simulink model "model"  (R2024a)
settings: Solver=VariableStepAuto  StartTime=0.0  StopTime=80  RelTol=1e-3
values from neighbouring files (symbols this model uses):
  b = 0.5*CdA*rho    (= 0.3316545)    [init.m]    (also in stateFcnTaycan.m)
  F_max = [22000 1710]    [init.m]    (also in stateFcnTaycan.m = interp1(v_to_F_max_lu, F_max_lu, v, 'linear'))
  F_min = -20000    [init.m]    (also in stateFcnTaycan.m)
  g = 9.81    [init.m]
  m = 2140    [init.m]    (also in stateFcnTaycan.m)
  Ts = 1    [init.m]
  v_to_F_max = [0 72]    [init.m]
libraries: simulink x3, mpclib x1
settings Model: Creator=berto  LastModifiedBy=berto

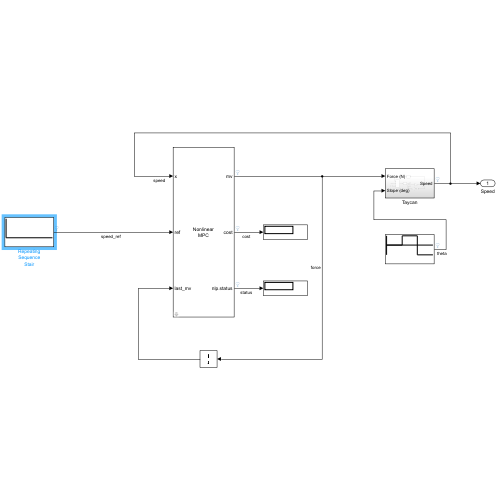
[thumbnail: Simulink's stored preview of the top-level diagram]
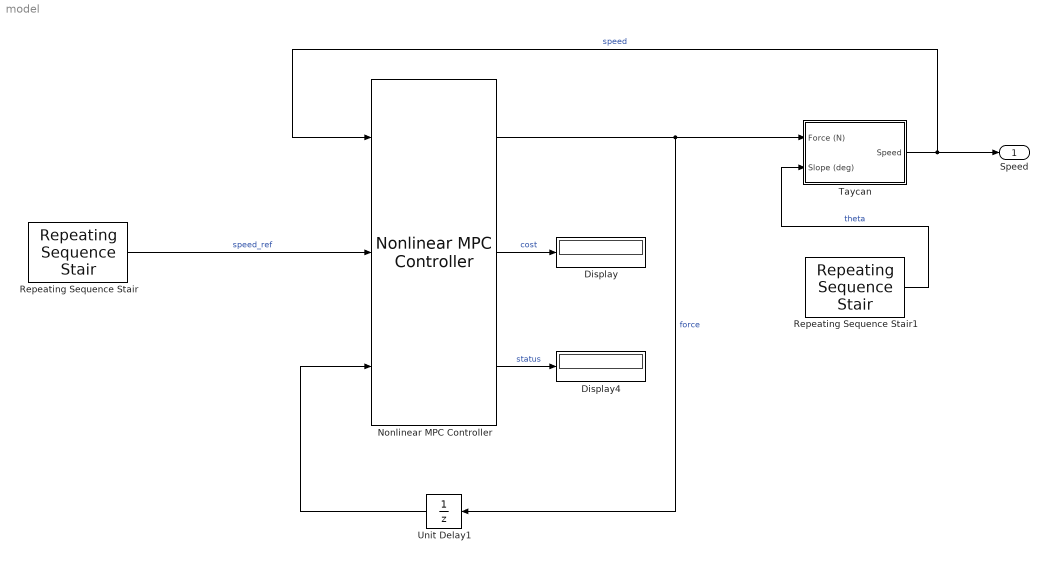
== system model ==
  Display : Display
  Display4 : Display
  Nonlinear MPC Controller : mpclib/Nonlinear MPC Controller  nlmpcobj=nlobj  UseObjectTs=on  UseMEX=off  md_enabled=off  mvtarget_enabled=off  param_enabled=off  cost_enabled=on  mvseq_enabled=off  stateseq_enabled=off  ovseq_enabled=off  slack_enabled=off  status_enabled=on  ov_min=off  ov_max=off  mv_min=off  mv_max=off  mvrate_min=off  mvrate_max=off  state_min=off  state_max=off  ov_weight=off  mv_weight=off  mvrate_weight=off  ecr_weight=off  nlp_initialize=off
  Repeating Sequence Stair : simulink/Sources/Repeating Sequence Stair  OutValues=40  tsamp=20  OutMin=[]  OutMax=[]  OutDataTypeStr=double  OutputDataTypeScalingMode=double  OutDataType=fixdt(0,8)  ConRadixGroup=Best Precision: Vector-wise  OutScaling=2^-12
  Repeating Sequence Stair1 : simulink/Sources/Repeating Sequence Stair  OutValues=[0 10 -10].'  tsamp=20  OutMin=[]  OutMax=[]  OutDataTypeStr=double  OutputDataTypeScalingMode=double  OutDataType=fixdt(0,8)  ConRadixGroup=Best Precision: Vector-wise  OutScaling=2^-12
  Taycan : Subsystem
  Unit Delay1 : UnitDelay  SampleTime=Ts  HasFrameUpgradeWarning=on
  Speed : Outport
  wires:
  Taycan/1(Speed) -> Nonlinear MPC Controller/1, Speed/1  "speed"
  Nonlinear MPC Controller/1 -> Taycan/1(Force (N)), Unit Delay1/1  "force"
  Repeating Sequence Stair/1 -> Nonlinear MPC Controller/2  "speed_ref"
  Unit Delay1/1 -> Nonlinear MPC Controller/3
  Nonlinear MPC Controller/2 -> Display/1  "cost"
  Nonlinear MPC Controller/3 -> Display4/1  "status"
  Repeating Sequence Stair1/1 -> Taycan/2(Slope (deg))  "theta"

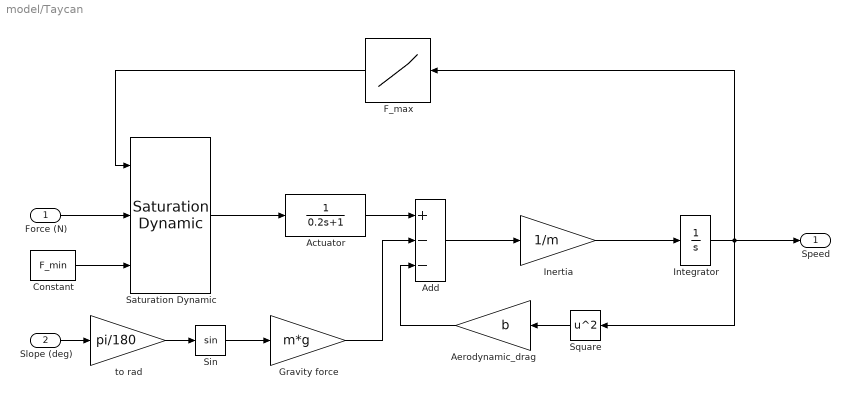
== system model/Taycan ==
  Force (N) : Inport
  Slope (deg) : Inport  Port=2
  Actuator : TransferFcn  Denominator=[0.2 1]
  Add : Sum  Inputs=+--
  Aerodynamic_drag : Gain  Gain=b
  Constant : Constant  Value=F_min
  F_max : Lookup_n-D  NumberOfTableDimensions=1  BreakpointsForDimension1=v_to_F_max  Table=F_max  ExtrapMethod=Clip  InternalRulePriority=Speed  RndMeth=Simplest
  Gravity force : Gain  Gain=m*g
  Inertia : Gain  Gain=1/m
  Integrator : Integrator
  Saturation Dynamic : simulink/Discontinuities/Saturation Dynamic  OutMin=[]  OutMax=[]  OutDataTypeStr=Inherit: Same as second input  OutDataType=fixdt(1, 16)  OutScaling=2^-10  DoSatur=off
  Sin : Trigonometry
  Square : Math  Operator=square
  to rad : Gain  Gain=pi/180
  Speed : Outport
  wires:
  Force (N)/1 -> Saturation Dynamic/2
  Actuator/1 -> Add/1
  Integrator/1 -> F_max/1, Speed/1, Square/1
  Constant/1 -> Saturation Dynamic/3
  Saturation Dynamic/1 -> Actuator/1
  F_max/1 -> Saturation Dynamic/1
  Aerodynamic_drag/1 -> Add/3
  Add/1 -> Inertia/1
  Inertia/1 -> Integrator/1
  Square/1 -> Aerodynamic_drag/1
  Slope (deg)/1 -> to rad/1
  Sin/1 -> Gravity force/1
  Gravity force/1 -> Add/2
  to rad/1 -> Sin/1
